simulink model "FLC_PBESS_V1"  (R2021a)
settings: Solver=ode23  StartTime=0.0  StopTime=3600*24  RelTol=1e-3
undefined symbols (not defined in the file or in its folder): f_serv_low, f_serv_upp, initSOC_BES, Ion, Lithium, Npar, Nser, P_serv_low, P_serv_upp, RatedPower
libraries: spsBatteryLib x2, spsControlledCurrentSourceLib x2, spspowerguiLib x2, fuzblock x2
settings Model: SimulationMode=accelerator  Creator=Sergio Cantillo  LastModifiedBy=Sergio Cantillo
settings DataIOCC: SaveTime=off  ReturnWorkspaceOutputs=off

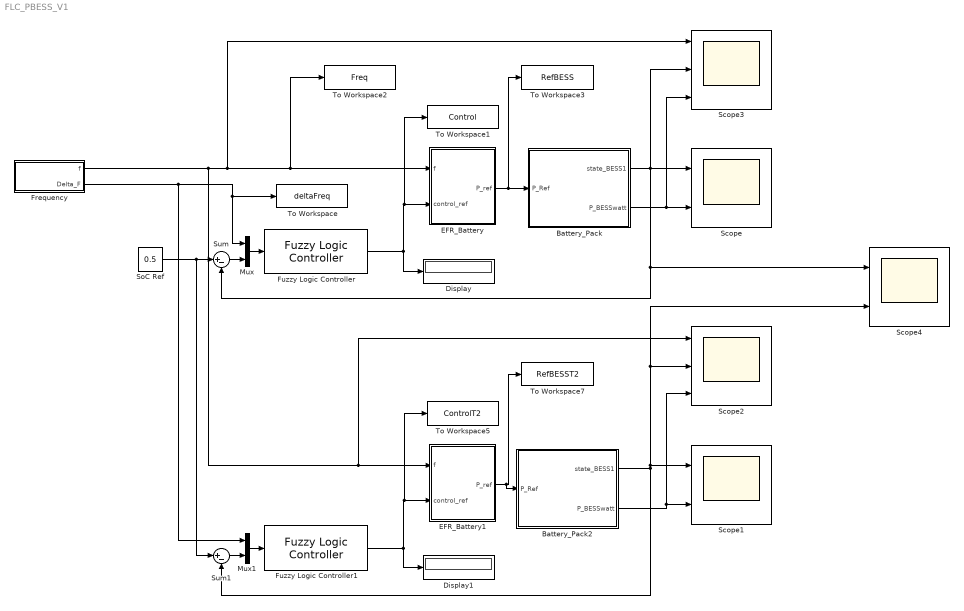
== system FLC_PBESS_V1 ==
  Battery_Pack : Subsystem
  Battery_Pack2 : Subsystem
  Display : Display
  Display1 : Display
  EFR_Battery : Subsystem
  EFR_Battery1 : Subsystem
  Frequency : Subsystem
  Fuzzy Logic Controller : fuzblock/Fuzzy Logic  Controller  FIS=FLCEFR  OutputSampleNumber=101  DataType=double  FuzzifiedInputs=off  RuleFiringStrengths=off  RuleOutputs=off  AggregatedOutputs=off  SimulateUsing=Interpreted execution  OutOfRangeInputValueMessage=warning  NoRuleFiredMessage=warning  EmptyOutputFuzzySetMessage=warning
  Fuzzy Logic Controller1 : fuzblock/Fuzzy Logic  Controller  FIS=FLCEFR_T2  OutputSampleNumber=101  DataType=double  FuzzifiedInputs=off  RuleFiringStrengths=off  RuleOutputs=off  AggregatedOutputs=off  SimulateUsing=Interpreted execution  OutOfRangeInputValueMessage=warning  NoRuleFiredMessage=warning  EmptyOutputFuzzySetMessage=warning
  Mux : Mux  Inputs=2
  Mux1 : Mux  Inputs=2
  Scope : Scope  NumInputPorts=2
  Scope1 : Scope  NumInputPorts=2
  Scope2 : Scope  NumInputPorts=3
  Scope3 : Scope  NumInputPorts=3
  Scope4 : Scope  NumInputPorts=2
  SoC Ref : Constant  Value=0.5
  Sum : Sum  Inputs=|+-
  Sum1 : Sum  Inputs=|+-
  To Workspace : ToWorkspace  VariableName=deltaFreq  SampleTime=-1
  To Workspace1 : ToWorkspace  VariableName=Control  SampleTime=-1
  To Workspace2 : ToWorkspace  VariableName=Freq  SampleTime=-1
  To Workspace3 : ToWorkspace  VariableName=RefBESS  SampleTime=-1
  To Workspace5 : ToWorkspace  VariableName=ControlT2  SampleTime=-1
  To Workspace7 : ToWorkspace  VariableName=RefBESST2  SampleTime=-1
  wires:
  EFR_Battery/1(P_ref) -> To Workspace3/1, Battery_Pack/1(P_Ref)
  Battery_Pack/1(state_BESS1) -> Scope3/2, Scope4/1, Sum/2, Scope/1
  Fuzzy Logic Controller/1 -> Display/1, To Workspace1/1, EFR_Battery/2(control_ref)
  Mux/1 -> Fuzzy Logic Controller/1
  Frequency/2(Delta_F) -> Mux1/1, Mux/1, To Workspace/1
  SoC Ref/1 -> Sum1/1, Sum/1
  Sum/1 -> Mux/2
  Battery_Pack/2(P_BESSwatt) -> Scope3/3, Scope/2
  Frequency/1(f) -> Scope2/1, EFR_Battery1/1(f), Scope3/1, To Workspace2/1, EFR_Battery/1(f)
  Fuzzy Logic Controller1/1 -> Display1/1, To Workspace5/1, EFR_Battery1/2(control_ref)
  Battery_Pack2/1(state_BESS1) -> Scope4/2, Scope2/2, Scope1/1, Sum1/2
  Battery_Pack2/2(P_BESSwatt) -> Scope2/3, Scope1/2
  Sum1/1 -> Mux1/2
  EFR_Battery1/1(P_ref) -> To Workspace7/1, Battery_Pack2/1(P_Ref)
  Mux1/1 -> Fuzzy Logic Controller1/1

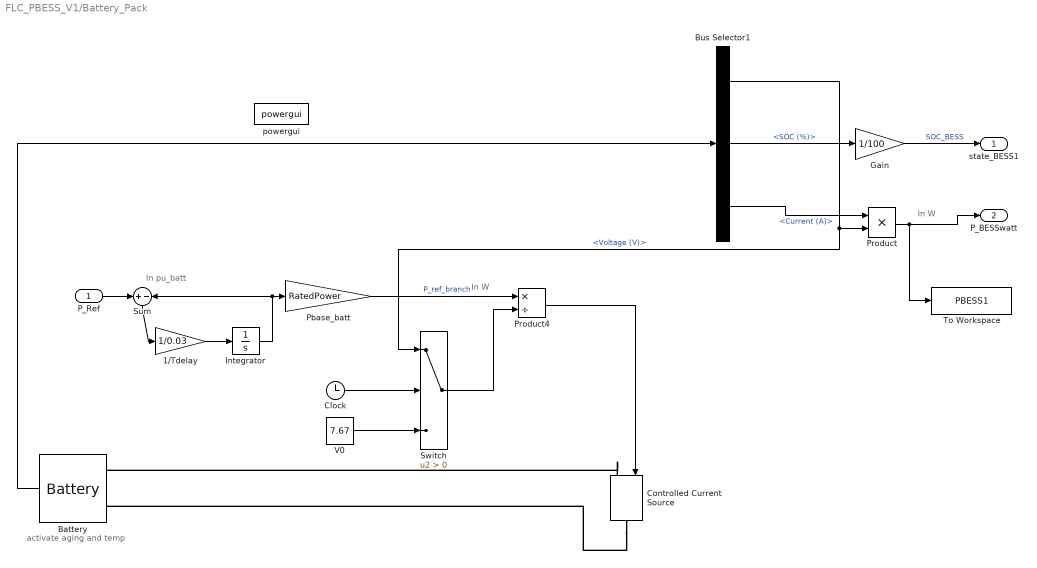
== system FLC_PBESS_V1/Battery_Pack ==
  note: activate aging and temp
  note: In W
  note: In pu_batt
  note: In W
  P_Ref : Inport
  1/Tdelay : Gain  Gain=1/0.03
  Battery : spsBatteryLib/Battery  BatType=Lithium-Ion  ShowTempParam=off  ThermalPreset=no  ShowAgeParam=off  NomV=7.2*Nser  NomQ=5.5*Npar  SOC=initSOC_BES*100  Batt_Tr=1  PresetModel=off  MaxQ=5.5*Npar  MinV=5400  FullV=8.3807*Nser  Dis_rate=2.3913*Npar  R=0.013091*Nser/Npar  Normal_OP=4.9739*Npar  expZone="[7.7788*Nser     0.27022*Npar]"  current=[5.4 21.6 32.5]  Units=Time  Tci=20  NomT=20  T2=-30  MaxQ2=4.8  FullV2=7.1  Normal_OP2=5.655  expZone2="[6.58           1]"  Rca=0.6  ti=2000  Dp=0  Neq0=0  Tsim=1e6  Ta1=25  Qeol=5.4*0.9  Reol=0.013333*1.2  Char_age=[2.3478, 3]  Dis_age=[2.3478, 10]  N1=1500  N2=10500  N3=1000  N4=1400  Ta2=45  N5=950
  Bus Selector1 : BusSelector  OutputSignals=Voltage (V),SOC (%),Current (A)
  Clock : Clock
  Controlled Current Source : spsControlledCurrentSourceLib/Controlled Current Source  Initialize=off  Source_Type=DC  Amplitude=20  Phase=0  Frequency=0  Measurements=None
  Gain : Gain  Gain=1/100
  Integrator : Integrator
  Pbase_batt : Gain  Gain=RatedPower
  Product : Product
  Product4 : Product  Inputs=*/
  Sum : Sum  Inputs=+-
  Switch : Switch  Criteria=u2 > Threshold
  To Workspace : ToWorkspace  VariableName=PBESS1  SampleTime=1
  V0 : Constant  Value=7.67
  powergui : spspowerguiLib/powergui  SimulationMode=Discrete  SampleTime=1  frequency=60  Iterations=50  frequencyindice=0  Pbase=100e6  ErrMax=1e-4  UnitsV=kV  UnitsW=MW  buscounter=0  FunctionMessages=off  echomessages=off  EnableUseOfTLC=off  CurrentSourceSwitches=off  DisableSnubberDevices=off  DisableRonSwitches=off  DisableVfSwitches=off  DisplayEquations=off  AutomaticDiscreteSolvers=off  SolverType=Tustin  Interpol=off  ExternalGateDelay=off  methode=off  Ts=0  x0status=blocks  SPID=off  SwTol=0  HookPort=off  NonlinearTolerance=1e-4  nMaxIteration=100  ContinueOnMaxIteration=off  RestoreLinks=warning  ResistiveCurrentMeasurement=off  Frange=[0:2:500]  Ylog=off  Xlog=on  ShowGrid=off  save=off  variable=ZData  structure=0  ZoomFFT=on  StartTime=0.0  cycles=1  DisplayStyle=1  fundamental=60  FreqAxis=off  MaxFrequency=1000  frequencyindicesteady=1  RmsSteady=1  display=off
  state_BESS1 : Outport  VectorParamsAs1DForOutWhenUnconnected=off
  P_BESSwatt : Outport  Port=2  VectorParamsAs1DForOutWhenUnconnected=off
  wires:
  Bus Selector1/1 -> Switch/1, Product/2  "<Voltage (V)>"
  Bus Selector1/2 -> Gain/1  "<SOC (%)>"
  Battery/1 -> Bus Selector1/1
  Bus Selector1/3 -> Product/1  "<Current (A)>"
  Gain/1 -> state_BESS1/1  "SOC_BESS"
  V0/1 -> Switch/3
  Pbase_batt/1 -> Product4/1  "P_ref_branch"
  Clock/1 -> Switch/2
  Product4/1 -> Controlled Current Source/1
  Switch/1 -> Product4/2
  1/Tdelay/1 -> Integrator/1
  P_Ref/1 -> Sum/1
  Sum/1 -> 1/Tdelay/1
  Integrator/1 -> Sum/2, Pbase_batt/1
  Product/1 -> To Workspace/1, P_BESSwatt/1
  connections:
  Controlled Current Source/RConn1 -- Battery/LConn2
  Controlled Current Source/LConn1 -- Battery/LConn1

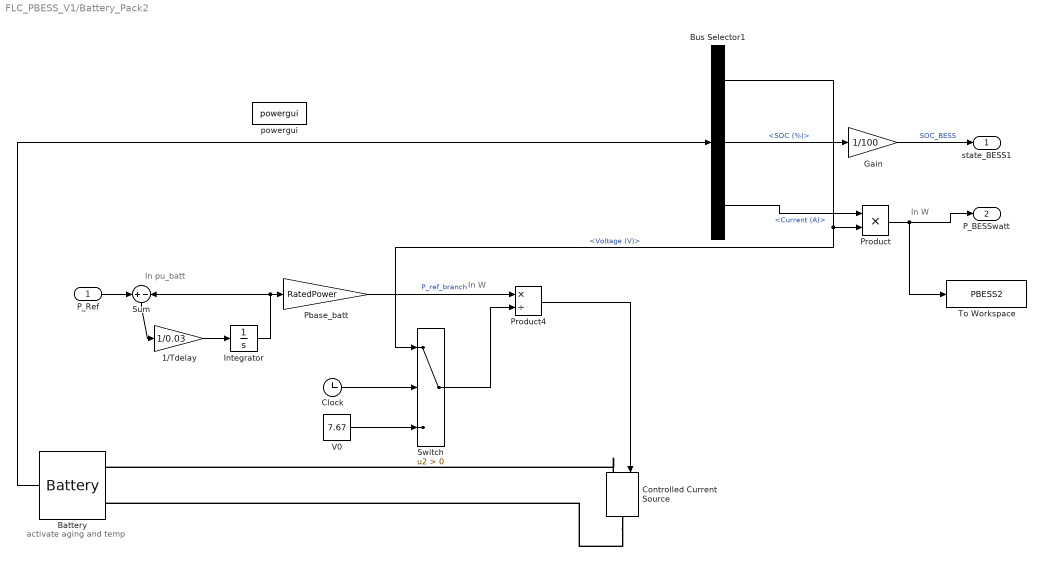
== system FLC_PBESS_V1/Battery_Pack2 ==
  note: activate aging and temp
  note: In W
  note: In pu_batt
  note: In W
  P_Ref : Inport
  1/Tdelay : Gain  Gain=1/0.03
  Battery : spsBatteryLib/Battery  BatType=Lithium-Ion  ShowTempParam=off  ThermalPreset=no  ShowAgeParam=off  NomV=7.2*Nser  NomQ=5.5*Npar  SOC=initSOC_BES*100  Batt_Tr=1  PresetModel=off  MaxQ=5.5*Npar  MinV=5400  FullV=8.3807*Nser  Dis_rate=2.3913*Npar  R=0.013091*Nser/Npar  Normal_OP=4.9739*Npar  expZone="[7.7788*Nser     0.27022*Npar]"  current=[5.4 21.6 32.5]  Units=Time  Tci=20  NomT=20  T2=-30  MaxQ2=4.8  FullV2=7.1  Normal_OP2=5.655  expZone2="[6.58           1]"  Rca=0.6  ti=2000  Dp=0  Neq0=0  Tsim=1e6  Ta1=25  Qeol=5.4*0.9  Reol=0.013333*1.2  Char_age=[2.3478, 3]  Dis_age=[2.3478, 10]  N1=1500  N2=10500  N3=1000  N4=1400  Ta2=45  N5=950
  Bus Selector1 : BusSelector  OutputSignals=Voltage (V),SOC (%),Current (A)
  Clock : Clock
  Controlled Current Source : spsControlledCurrentSourceLib/Controlled Current Source  Initialize=off  Source_Type=DC  Amplitude=20  Phase=0  Frequency=0  Measurements=None
  Gain : Gain  Gain=1/100
  Integrator : Integrator
  Pbase_batt : Gain  Gain=RatedPower
  Product : Product
  Product4 : Product  Inputs=*/
  Sum : Sum  Inputs=+-
  Switch : Switch  Criteria=u2 > Threshold
  To Workspace : ToWorkspace  VariableName=PBESS2  SampleTime=1
  V0 : Constant  Value=7.67
  powergui : spspowerguiLib/powergui  SimulationMode=Discrete  SampleTime=1  frequency=60  Iterations=50  frequencyindice=0  Pbase=100e6  ErrMax=1e-4  UnitsV=kV  UnitsW=MW  buscounter=0  FunctionMessages=off  echomessages=off  EnableUseOfTLC=off  CurrentSourceSwitches=off  DisableSnubberDevices=off  DisableRonSwitches=off  DisableVfSwitches=off  DisplayEquations=off  AutomaticDiscreteSolvers=off  SolverType=Tustin  Interpol=off  ExternalGateDelay=off  methode=off  Ts=0  x0status=blocks  SPID=off  SwTol=0  HookPort=off  NonlinearTolerance=1e-4  nMaxIteration=100  ContinueOnMaxIteration=off  RestoreLinks=warning  ResistiveCurrentMeasurement=off  Frange=[0:2:500]  Ylog=off  Xlog=on  ShowGrid=off  save=off  variable=ZData  structure=0  ZoomFFT=on  StartTime=0.0  cycles=1  DisplayStyle=1  fundamental=60  FreqAxis=off  MaxFrequency=1000  frequencyindicesteady=1  RmsSteady=1  display=off
  state_BESS1 : Outport  VectorParamsAs1DForOutWhenUnconnected=off
  P_BESSwatt : Outport  Port=2  VectorParamsAs1DForOutWhenUnconnected=off
  wires:
  Bus Selector1/1 -> Switch/1, Product/2  "<Voltage (V)>"
  Bus Selector1/2 -> Gain/1  "<SOC (%)>"
  Battery/1 -> Bus Selector1/1
  Bus Selector1/3 -> Product/1  "<Current (A)>"
  Gain/1 -> state_BESS1/1  "SOC_BESS"
  V0/1 -> Switch/3
  Pbase_batt/1 -> Product4/1  "P_ref_branch"
  Clock/1 -> Switch/2
  Product4/1 -> Controlled Current Source/1
  Switch/1 -> Product4/2
  1/Tdelay/1 -> Integrator/1
  P_Ref/1 -> Sum/1
  Sum/1 -> 1/Tdelay/1
  Integrator/1 -> Sum/2, Pbase_batt/1
  Product/1 -> To Workspace/1, P_BESSwatt/1
  connections:
  Controlled Current Source/RConn1 -- Battery/LConn2
  Controlled Current Source/LConn1 -- Battery/LConn1

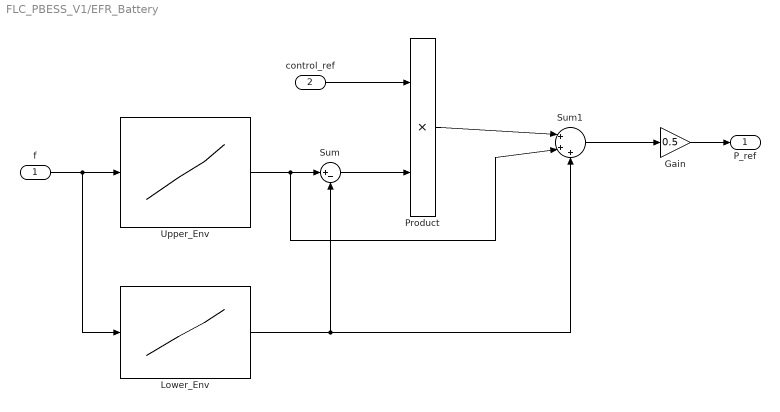
== system FLC_PBESS_V1/EFR_Battery ==
  f : Inport
  control_ref : Inport  Port=2  SampleTime=10
  Gain : Gain  Gain=0.5
  Lower_Env : Lookup_n-D  NumberOfTableDimensions=1  BreakpointsForDimension1=f_serv_low  Table=P_serv_low  ExtrapMethod=Clip  UseLastTableValue=on  InternalRulePriority=Speed  RndMeth=Simplest  InputSameDT=on
  Product : Product
  Sum : Sum  Inputs=|+-
  Sum1 : Sum  Inputs=|+++
  Upper_Env : Lookup_n-D  NumberOfTableDimensions=1  BreakpointsForDimension1=f_serv_upp  Table=P_serv_upp  ExtrapMethod=Clip  UseLastTableValue=on  InternalRulePriority=Speed  RndMeth=Simplest  InputSameDT=on
  P_ref : Outport  VectorParamsAs1DForOutWhenUnconnected=off
  wires:
  f/1 -> Lower_Env/1, Upper_Env/1
  control_ref/1 -> Product/1
  Lower_Env/1 -> Sum1/3, Sum/2
  Gain/1 -> P_ref/1
  Sum/1 -> Product/2
  Product/1 -> Sum1/1
  Sum1/1 -> Gain/1
  Upper_Env/1 -> Sum/1, Sum1/2

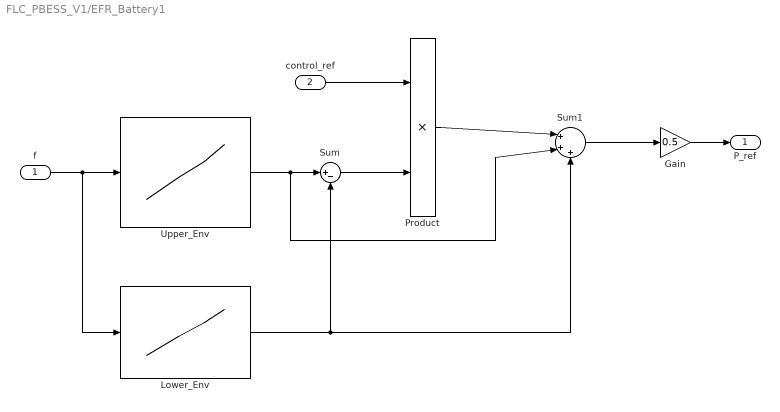
== system FLC_PBESS_V1/EFR_Battery1 ==
  f : Inport
  control_ref : Inport  Port=2  SampleTime=10
  Gain : Gain  Gain=0.5
  Lower_Env : Lookup_n-D  NumberOfTableDimensions=1  BreakpointsForDimension1=f_serv_low  Table=P_serv_low  ExtrapMethod=Clip  UseLastTableValue=on  InternalRulePriority=Speed  RndMeth=Simplest  InputSameDT=on
  Product : Product
  Sum : Sum  Inputs=|+-
  Sum1 : Sum  Inputs=|+++
  Upper_Env : Lookup_n-D  NumberOfTableDimensions=1  BreakpointsForDimension1=f_serv_upp  Table=P_serv_upp  ExtrapMethod=Clip  UseLastTableValue=on  InternalRulePriority=Speed  RndMeth=Simplest  InputSameDT=on
  P_ref : Outport  VectorParamsAs1DForOutWhenUnconnected=off
  wires:
  f/1 -> Lower_Env/1, Upper_Env/1
  control_ref/1 -> Product/1
  Lower_Env/1 -> Sum1/3, Sum/2
  Gain/1 -> P_ref/1
  Sum/1 -> Product/2
  Product/1 -> Sum1/1
  Sum1/1 -> Gain/1
  Upper_Env/1 -> Sum/1, Sum1/2

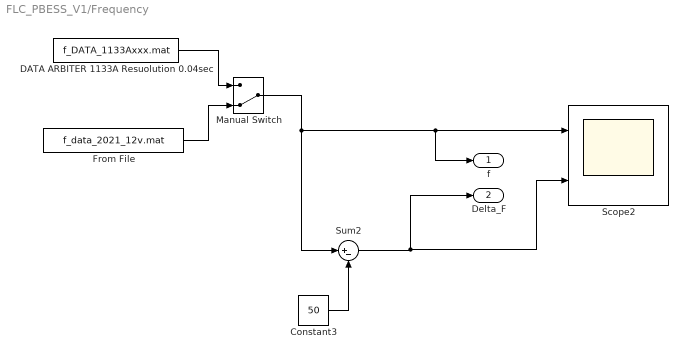
== system FLC_PBESS_V1/Frequency ==
  Constant3 : Constant  Value=50
  "DATA ARBITER 1133A Resuolution 0.04sec " : FromFile  FileName=f_DATA_1133Axxx.mat
  From File : FromFile  FileName=f_data_2021_12v.mat  ExtrapolationBeforeFirstDataPoint=Ground value
  Manual Switch : ManualSwitch  CurrentSetting=0
  Scope2 : Scope  NumInputPorts=2
  Sum2 : Sum  Inputs=|+-
  f : Outport
  Delta_F : Outport  Port=2
  wires:
  Constant3/1 -> Sum2/2
  Sum2/1 -> Scope2/2, Delta_F/1
  From File/1 -> Manual Switch/2
  Manual Switch/1 -> f/1, Scope2/1, Sum2/1
  "DATA ARBITER 1133A Resuolution 0.04sec "/1 -> Manual Switch/1
